simulink model "Simulation_Fahrmodell_v3_straight_line_R2024b"  (R2024b)
settings: Solver=ode14x  StartTime=0.0  StopTime=600  FixedStep=0.005  RelTol=1e-3
values from neighbouring files (symbols this model uses):
  bat = bat.computePack()    [DoE_main.m]    (also in DoE_main_sensitivity.m)
  cp = cp.computeP4Map(val_P4, 0, val_P4_DM, 0, 0)    [DoE_main.m]    (also in DoE_main_sensitivity.m = cp.computeP4Map(P4, E2, P4_DM, E3, E4))
  gb = gb.computeShiftMaps()    [DoE_main.m]    (also in DoE_main_sensitivity.m)
  P4 = cfgNum(cfg, 'P4', 0)    [DoE_main_sensitivity.m]    (also in PowertrainConfig.m = 0)
  P4_DM = cfgNum(cfg, 'P4_DM', 0)    [DoE_main_sensitivity.m]    (also in PowertrainConfig.m = 0)
  pt = pt.setupHybrid()    [DoE_main.m]    (also in DoE_main_sensitivity.m)
  veh = VehicleConfig()    [DoE_main.m]    (also in DoE_main_sensitivity.m)
undefined symbols (not defined in the file or in its folder): cp_Zelle_JpkgK, Ice_derfacLoadDecrease_MAP, Ice_derfacLoadIncrease_MAP, Ice_n_axis, Ice_relLoadMax_CUR_n, Ice_relLoadMax_CUR_val, Ice_rl_axis_norm, seconds, SKO_STREET_CHAL, SKO_WHEEL_TYP_CHAL, slip_pacejka, T_init_degC, Track, TT_sliced, use_turbo_model, v_Fzg_init_kmph
libraries: nesl_utility x15, fl_lib x9, simulink x4
(part 1 of 6)
settings Model: Creator=TZ555AA  LastModifiedBy=SHIKHAR TAKKE
settings DebuggingCC: SignalInfNanChecking=warning
settings RTWCC: GPUComputeCapability=3.5

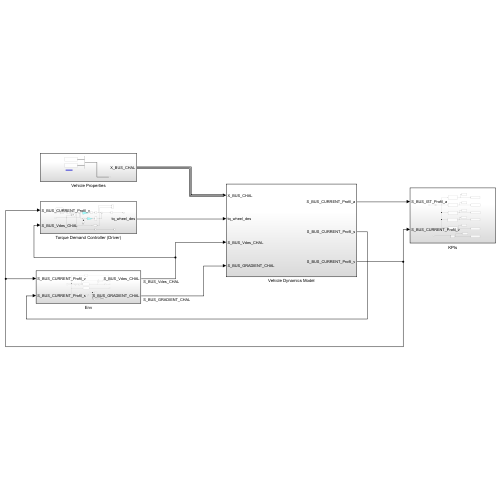
[thumbnail: Simulink's stored preview of the top-level diagram]
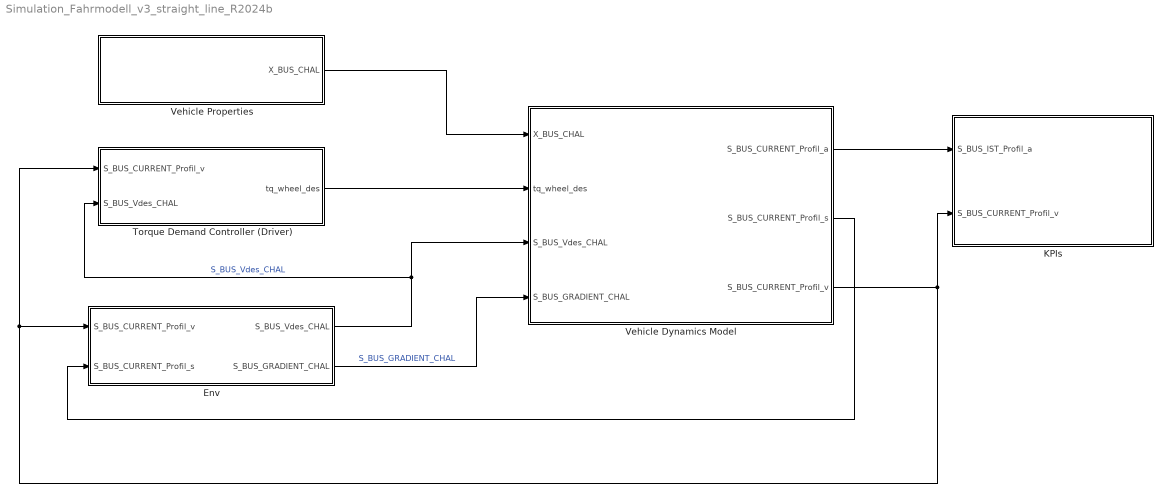
== system Simulation_Fahrmodell_v3_straight_line_R2024b ==
  Env : Subsystem
  KPIs : Subsystem
  Torque Demand Controller (Driver) : Subsystem
  "Vehicle Dynamics Model " : Subsystem
  Vehicle Properties : Subsystem
  wires:
  "Vehicle Dynamics Model "/1(S_BUS_CURRENT_Profil_a) -> KPIs/1(S_BUS_IST_Profil_a)
  "Vehicle Dynamics Model "/3(S_BUS_CURRENT_Profil_v) -> KPIs/2(S_BUS_CURRENT_Profil_v), Torque Demand Controller (Driver)/1(S_BUS_CURRENT_Profil_v), Env/1(S_BUS_CURRENT_Profil_v)
  "Vehicle Dynamics Model "/2(S_BUS_CURRENT_Profil_s) -> Env/2(S_BUS_CURRENT_Profil_s)
  Env/2(S_BUS_GRADIENT_CHAL) -> "Vehicle Dynamics Model "/4(S_BUS_GRADIENT_CHAL)  "S_BUS_GRADIENT_CHAL"
  Env/1(S_BUS_Vdes_CHAL) -> "Vehicle Dynamics Model "/3(S_BUS_Vdes_CHAL), Torque Demand Controller (Driver)/2(S_BUS_Vdes_CHAL)  "S_BUS_Vdes_CHAL"
  Torque Demand Controller (Driver)/1(tq_wheel_des) -> "Vehicle Dynamics Model "/2(tq_wheel_des)
  Vehicle Properties/1(X_BUS_CHAL) -> "Vehicle Dynamics Model "/1(X_BUS_CHAL)

== system Simulation_Fahrmodell_v3_straight_line_R2024b/Env ==
  S_BUS_CURRENT_Profil_v : Inport
  S_BUS_CURRENT_Profil_s : Inport  Port=2
  Bus Creator : BusCreator  Inputs=2
  Clock : Clock
  Constant : Constant  Value=seconds(TT_sliced.time(end))
  Display1 : Display
  Display3 : Display
  Gain : Gain
  Gain1 : Gain
  Gain2 : Gain  Gain=1/3.6
  Gain3 : Gain  Gain=3.6
  Gain4 : Gain
  Min : MinMax  Inputs=2
  Minus : Sum  Inputs=+-
  Nürburgring Simulation J. Siwig 469s (7m 49s) : Lookup_n-D  NumberOfTableDimensions=1  BreakpointsForDimension1=TT_sliced.s_m  Table=TT_sliced.v_Fzg_kmph  ExtrapMethod=Clip  UseLastTableValue=on  InternalRulePriority=Speed  RndMeth=Simplest
  Nürburgring Simulation J. Siwig 469s (7m 49s) time(s) : Lookup_n-D  NumberOfTableDimensions=1  BreakpointsForDimension1=TT_sliced.s_m  Table=seconds(TT_sliced.time)  ExtrapMethod=Clip  UseLastTableValue=on  InternalRulePriority=Speed  RndMeth=Simplest
  Nürburgring (M. Siesmann) : Subsystem
  Nürburgring (M. Siesmann) Steigung [deg] : Subsystem
  Scope : Scope  NumInputPorts=3
  Scope1 : Scope  NumInputPorts=2
  S_BUS_Vdes_CHAL : Outport
  S_BUS_GRADIENT_CHAL : Outport  Port=2
  wires:
  Gain3/1 -> Gain/1, Nürburgring (M. Siesmann)/2(v_ist_kmph)  "v_ist_kmph"
  Gain4/1 -> Gain3/1  "v_ist_mps"
  S_BUS_CURRENT_Profil_v/1 -> Gain4/1
  S_BUS_CURRENT_Profil_s/1 -> Nürburgring Simulation J. Siwig 469s (7m 49s)/1, Nürburgring (M. Siesmann)/1(s_m), Nürburgring Simulation J. Siwig 469s (7m 49s) time(s)/1, Nürburgring (M. Siesmann) Steigung [deg]/1(s_m)
  Nürburgring (M. Siesmann) Steigung [deg]/1(steigung_deg) -> S_BUS_GRADIENT_CHAL/1  "S_BUS_STEIGUNG_CHAL"
  Gain2/1 -> S_BUS_Vdes_CHAL/1
  Nürburgring (M. Siesmann)/1(v_soll_kmph) -> Gain2/1, Gain1/1  "[km/h]"
  Nürburgring Simulation J. Siwig 469s (7m 49s)/1 -> Scope/1  "MESSUNG v_Fzg_kmph"
  Gain/1 -> Scope/2  "SIM v_ist_kmph"
  Gain1/1 -> Scope/3  "SIM v_soll_kmph"
  Clock/1 -> Minus/2, Bus Creator/2, Display3/1  "SIM zeit"
  Min/1 -> Bus Creator/1, Minus/1, Display1/1  "MESSUNG zeit"
  Minus/1 -> Scope1/2  "DELTA zeit"
  Bus Creator/1 -> Scope1/1
  Constant/1 -> Min/2
  Nürburgring Simulation J. Siwig 469s (7m 49s) time(s)/1 -> Min/1  "MESSUNG zeit"

== system Simulation_Fahrmodell_v3_straight_line_R2024b/KPIs ==
  S_BUS_IST_Profil_a : Inport
  S_BUS_CURRENT_Profil_v : Inport  Port=2
  Display{1..5,7} (6 alike) : Display
  Gain : Gain  Gain=3.6
  MinMax Running Resettable1 : simulink/Math Operations/MinMax Running Resettable  Function=max  vinit=0
  To Workspace1 : ToWorkspace  VariableName=time_0_to_100  SampleTime=-1
      settings: MaxDataPoints=1
  To Workspace2 : ToWorkspace  VariableName=time_80_to_120  SampleTime=-1
      settings: MaxDataPoints=1
  To Workspace3 : ToWorkspace  VariableName=time_0_to_200  SampleTime=-1
      settings: MaxDataPoints=1
  To Workspace4 : ToWorkspace  VariableName=max_speed  SampleTime=-1
      settings: MaxDataPoints=1
  To Workspace5 : ToWorkspace  VariableName=max_launch_acc  SampleTime=-1
      settings: MaxDataPoints=1
  To Workspace6 : ToWorkspace  VariableName=time_60_to_120  SampleTime=-1
      settings: MaxDataPoints=1
  max speed : Subsystem
  time_0_to_100 : Subsystem
  time_0_to_200 : Subsystem
  time_60_to_120 : Subsystem
  time_80_to_120 : Subsystem
  wires:
  time_80_to_120/1(Out1) -> Display5/1, To Workspace2/1
  time_0_to_200/1(Out1) -> To Workspace3/1, Display4/1
  time_0_to_100/1(Out1) -> Display2/1, To Workspace1/1
  S_BUS_CURRENT_Profil_v/1 -> Gain/1
  S_BUS_IST_Profil_a/1 -> MinMax Running Resettable1/1
  MinMax Running Resettable1/1 -> Display7/1, To Workspace5/1
  max speed/1(u1) -> Display1/1, To Workspace4/1
  time_60_to_120/1(Out1) -> To Workspace6/1, Display3/1
  Gain/1 -> time_0_to_100/1(SIM v_ist_kmph), time_0_to_200/1(SIM v_ist_kmph), time_60_to_120/1(SIM v_ist_kmph), max speed/1(u), time_80_to_120/1(SIM v_ist_kmph)

== system Simulation_Fahrmodell_v3_straight_line_R2024b/Torque Demand Controller (Driver) ==
  S_BUS_CURRENT_Profil_v : Inport
  S_BUS_Vdes_CHAL : Inport  Port=2
  Drv_kmh2gradtqDriver_C Value: 300 : Gain  Gain=100
  Drv_kmh2tqDriver_C Value: 1500 : Gain  Gain=500
  Feedback I-Part at v=0 : Lookup_n-D  NumberOfTableDimensions=1  BreakpointsForDimension1="[-1 -0.0001  0  0.0001  1]"  Table="[0 0  1  0  0]"  InternalRulePriority=Speed  RndMeth=Simplest
  Gain : Gain
  Gain1 : Gain  Gain=0.005
  Gain2 : Gain  Gain=3.6
  Integrator : Integrator  LimitOutput=on  UpperSaturationLimit=2000  LowerSaturationLimit=-1200
  LowPass4Solver : TransferFcn  Denominator=[0.0001 1]
  MinMax : MinMax  Inputs=2
  Mux : Mux  Inputs=2
  Product : Product
  Saturation : Saturate  UpperLimit=7000  LowerLimit=-5000
  Saturation1 3000 : Saturate  UpperLimit=9000  LowerLimit=-5000
  Scope Ctrl. : Scope  NumInputPorts=2
  Scope kmh : Scope
  Sum : Sum  Inputs=|+-
  Sum1 : Sum  Inputs=|++
  Sum2 : Sum  Inputs=|+-
  Terminator : Terminator  Commented=on
  v_maxKmhEdr : Constant  Value=350
  tq_wheel_des : Outport  VectorParamsAs1DForOutWhenUnconnected=off
  wires:
  Mux/1 -> Scope kmh/1
  Gain2/1 -> MinMax/2
  MinMax/1 -> Gain/1, Sum/1, Mux/1  "Env_kmhVehDesLim"
  Gain1/1 -> Product/2  "Drv_kmhVehDesLim"
  Integrator/1 -> Gain1/1, Sum1/2, Scope Ctrl./2  "Drv_tqICtrlDrv[Nm]"
  Sum1/1 -> Saturation1 3000/1  "tqDrvWheelAxDesUnlim"
  S_BUS_Vdes_CHAL/1 -> Gain2/1
  Sum2/1 -> Drv_kmh2gradtqDriver_C Value: 300/1
  Saturation/1 -> Sum1/1, Scope Ctrl./1  "Drv_tqPCtrlDrv[Nm]"
  Feedback I-Part at v=0/1 -> Product/1
  v_maxKmhEdr/1 -> MinMax/1
  Sum/1 -> Sum2/1, Drv_kmh2tqDriver_C Value: 1500/1
  LowPass4Solver/1 -> Saturation/1
  Drv_kmh2tqDriver_C Value: 1500/1 -> LowPass4Solver/1
  S_BUS_CURRENT_Profil_v/1 -> Feedback I-Part at v=0/1, Sum/2, Mux/2
  Drv_kmh2gradtqDriver_C Value: 300/1 -> Integrator/1
  Saturation1 3000/1 -> tq_wheel_des/1  "tq_wheel_des"
  Product/1 -> Sum2/2
  Gain/1 -> Terminator/1  "Drv_kmhVehDesLim"

== system Simulation_Fahrmodell_v3_straight_line_R2024b/Vehicle Dynamics Model  ==
  X_BUS_CHAL : Inport
  tq_wheel_des : Inport  Port=2
  S_BUS_Vdes_CHAL : Inport  Port=3
  S_BUS_GRADIENT_CHAL : Inport  Port=4
  Bremsen : Subsystem
      mask Display: image('BremseVAHA_1.png');
  "Computation of Distance, Speed and Acceleration" : Subsystem
  Drivetrain : Subsystem
  Driving Resistance : Subsystem
  PI-Regler neu : Subsystem
  S_BUS_CURRENT_Profil_a : Outport
  S_BUS_CURRENT_Profil_s : Outport  Port=2
  S_BUS_CURRENT_Profil_v : Outport  Port=3
  wires:
  S_BUS_Vdes_CHAL/1 -> PI-Regler neu/1(S_BUS_Vdes_CHAL)
  X_BUS_CHAL/1 -> "Computation of Distance, Speed and Acceleration"/1(X_BUS_CHAL), Bremsen/1(X_BUS_CHAL), Drivetrain/2(X_BUS_CHAL1), Driving Resistance/1(X_BUS_CHAL)  "X_BUS_CHAL"
  S_BUS_GRADIENT_CHAL/1 -> Driving Resistance/3(BUS_STEIGUNG), Drivetrain/4(S_BUS_GRADIENT)
  Drivetrain/1(F_Lat_max (N)) -> "Computation of Distance, Speed and Acceleration"/2(F_Lat_max (N))  "F_Lat_max (N)"
  PI-Regler neu/1(Regelfaktor [-1 .. 1]) -> Drivetrain/1(Regelfaktor), Bremsen/2(Regelfaktor [-1 .. 1])
  "Computation of Distance, Speed and Acceleration"/1(S_BUS_IST_Profil_v) -> Driving Resistance/4(S_BUS_IST_Profil_v), Drivetrain/5(S_BUS_IST_Profil_v1), PI-Regler neu/2(S_BUS_IST_Profil_v), S_BUS_CURRENT_Profil_v/1  "S_BUS_IST_Profil_v"
  "Computation of Distance, Speed and Acceleration"/2(S_BUS_IST_Profil_s) -> S_BUS_CURRENT_Profil_s/1
  "Computation of Distance, Speed and Acceleration"/3(S_BUS_IST_Profil_a) -> Drivetrain/6(S_BUS_IST_Profil_a1), Driving Resistance/5(S_BUS_IST_Profil_a), S_BUS_CURRENT_Profil_a/1
  Bremsen/1(Bremskraft (N)) -> "Computation of Distance, Speed and Acceleration"/4(Bremskraft (N))  "Bremskraft (N)"
  tq_wheel_des/1 -> Drivetrain/3(tq_wheel_des)
  Drivetrain/2(M_m_Nm) -> Driving Resistance/2(M_m_Nm)
  Driving Resistance/1(FW_RSV (N)) -> "Computation of Distance, Speed and Acceleration"/3(FW_RSV (N))

== system Simulation_Fahrmodell_v3_straight_line_R2024b/Vehicle Properties ==
  note: Vehicle characteristics
  Bus Creator : BusCreator  Inputs=2
  Fzg.-Eigenschaften : Subsystem
  Systemkonstanten : Subsystem
  X_BUS_CHAL : Outport
  wires:
  Fzg.-Eigenschaften/1(M_BUS_EIG_CHAL) -> Bus Creator/2  "M_BUS_EIG_CHAL"
  Bus Creator/1 -> X_BUS_CHAL/1  "X_BUS_CHAL"
  Systemkonstanten/1(M_BUS_SKO) -> Bus Creator/1  "M_BUS_SKO"

== system Simulation_Fahrmodell_v3_straight_line_R2024b/Env/Nürburgring (M. Siesmann) ==
  s_m : Inport
  v_ist_kmph : Inport  Port=2
  Constant1 : Constant  Value=Track.RoundOnly.s_cum__m(end)
  Constant15 : Constant  Value=10000
  Display3 : Display
  Display4 : Display
  Fahrdynamik: Kurvenradius und Querbeschleunigung : Subsystem
  Fahrdynamik: Sollgeschwindigkeit (Kamm'scher Kreis) : Subsystem
  Low Pass Filter Amplitude = 1 Cut Off Freq = 3 KHz : TransferFcn  Commented=through  Denominator=[1/(2*pi*3000) 1]
  Min : MinMax  Inputs=2
  Relational Operator1 : RelationalOperator  OutDataTypeStr=boolean  RndMeth=Simplest  InputSameDT=off
  Scope : Scope  NumInputPorts=3
  Stop Simulation : Stop
  v max min : Subsystem
  vMax__km_per_h(s) vMax_Fwd : Lookup_n-D  Commented=on  NumberOfTableDimensions=1  BreakpointsForDimension1=Track.RoundOnly.s_cum__m  Table=Track.RoundOnly.vMax__km_per_h  InternalRulePriority=Speed  RndMeth=Simplest
  vMax__km_per_h(s) vMax_Fwd1 : Lookup_n-D  NumberOfTableDimensions=1  BreakpointsForDimension1=[0,2000]  Table=[300,300]  InternalRulePriority=Speed  RndMeth=Simplest
  v_soll_kmph : Outport
  wires:
  v_ist_kmph/1 -> Fahrdynamik: Kurvenradius und Querbeschleunigung/1(v_ist_kmph), Fahrdynamik: Sollgeschwindigkeit (Kamm'scher Kreis)/1(v_ist_kmph)
  Fahrdynamik: Sollgeschwindigkeit (Kamm'scher Kreis)/1(v_soll_kmph) -> Low Pass Filter Amplitude = 1 Cut Off Freq = 3 KHz/1
  Fahrdynamik: Kurvenradius und Querbeschleunigung/1(a_y_ist_mps2) -> Fahrdynamik: Sollgeschwindigkeit (Kamm'scher Kreis)/2(a_y_ist_mps2)
  Relational Operator1/1 -> Stop Simulation/1
  Constant15/1 -> Display4/1, Relational Operator1/2
  Min/1 -> v max min/1(In1), Scope/3  "v_soll_kmph END"
  Fahrdynamik: Kurvenradius und Querbeschleunigung/2(r_kurven_m) -> Fahrdynamik: Sollgeschwindigkeit (Kamm'scher Kreis)/3(r_kurven_m)
  v max min/1(Out1) -> v_soll_kmph/1
  s_m/1 -> vMax__km_per_h(s) vMax_Fwd1/1, Fahrdynamik: Kurvenradius und Querbeschleunigung/2(s_m), Display3/1, Relational Operator1/1
  Low Pass Filter Amplitude = 1 Cut Off Freq = 3 KHz/1 -> Scope/2, Min/2  "v_soll_kmph FDyn"
  vMax__km_per_h(s) vMax_Fwd1/1 -> Min/1, Scope/1  "v_soll_kmph 3SIM"

== system Simulation_Fahrmodell_v3_straight_line_R2024b/Env/Nürburgring (M. Siesmann) Steigung [deg] ==
  s_m : Inport
  Agl_Elevation__deg(s_cum_m) : Lookup_n-D  Commented=on  NumberOfTableDimensions=1  BreakpointsForDimension1=Track.RoundOnly.s_cum__m  Table=Track.RoundOnly.Agl_Elevation__deg  InternalRulePriority=Speed  RndMeth=Simplest
  Agl_Elevation__deg(s_cum_m)1 : Lookup_n-D  NumberOfTableDimensions=1  BreakpointsForDimension1=[0,2000]  Table=[0,0]  InternalRulePriority=Speed  RndMeth=Simplest
  steigung_deg : Outport
  wires:
  Agl_Elevation__deg(s_cum_m)1/1 -> steigung_deg/1  "steigung_deg"
  s_m/1 -> Agl_Elevation__deg(s_cum_m)1/1

== system Simulation_Fahrmodell_v3_straight_line_R2024b/KPIs/max speed ==
  u : Inport
  R : Inport  Port=2
  Add : Sum  Inputs=+-
  Compare To Constant : simulink/Logic and Bit Operations/Compare To Constant  relop===  const=0  OutDataTypeStr=boolean
  Compare To Constant1 : simulink/Logic and Bit Operations/Compare To Constant  relop=>  const=35  OutDataTypeStr=boolean
  Constant : Constant
  Delay : Delay  InitialCondition=0
  Display6 : Display
  MinMax Running Resettable : simulink/Math Operations/MinMax Running Resettable  Function=max  vinit=0
  Stop Simulation : Stop
  Switch : Switch  Criteria=u2 > Threshold  SaturateOnIntegerOverflow=off  InputSameDT=off
  u1 : Outport
  wires:
  MinMax Running Resettable/1 -> Compare To Constant1/1, Add/1, Delay/1, u1/1
  Compare To Constant/1 -> Stop Simulation/1, Display6/1
  Delay/1 -> Switch/1
  Compare To Constant1/1 -> Switch/2
  Add/1 -> Compare To Constant/1
  Constant/1 -> Switch/3
  Switch/1 -> Add/2
  u/1 -> MinMax Running Resettable/1
  R/1 -> MinMax Running Resettable/2

== system Simulation_Fahrmodell_v3_straight_line_R2024b/KPIs/time_0_to_100 ==
  SIM v_ist_kmph : Inport
  Clock : Clock
      settings: Decimation=100
  Constant : Constant
  Constant1 : Constant  Value=0
  Switch : Switch  Threshold=100  SaturateOnIntegerOverflow=off  InputSameDT=off
  Triggered Subsystem : Subsystem  TreatAsAtomicUnit=on
  Out1 : Outport
  wires:
  Constant/1 -> Switch/1
  SIM v_ist_kmph/1 -> Switch/2
  Switch/1 -> Triggered Subsystem/Trigger
  Clock/1 -> Triggered Subsystem/1(In1)
  Constant1/1 -> Switch/3
  Triggered Subsystem/1(Out1) -> Out1/1

== system Simulation_Fahrmodell_v3_straight_line_R2024b/KPIs/time_0_to_200 ==
  SIM v_ist_kmph : Inport
  Clock : Clock
      settings: Decimation=100
  Constant : Constant
  Constant1 : Constant  Value=0
  Switch : Switch  Threshold=200  SaturateOnIntegerOverflow=off  InputSameDT=off
  Triggered Subsystem : Subsystem  TreatAsAtomicUnit=on
  Out1 : Outport
  wires:
  Triggered Subsystem/1(Out1) -> Out1/1
  Constant1/1 -> Switch/3
  Clock/1 -> Triggered Subsystem/1(In1)
  Switch/1 -> Triggered Subsystem/Trigger
  SIM v_ist_kmph/1 -> Switch/2
  Constant/1 -> Switch/1

== system Simulation_Fahrmodell_v3_straight_line_R2024b/KPIs/time_60_to_120 ==
  SIM v_ist_kmph : Inport
  Add : Sum  Inputs=+-
  time_0_to_120 : Subsystem
  time_0_to_60 : Subsystem
  Out1 : Outport
  wires:
  Add/1 -> Out1/1
  time_0_to_120/1(Out1) -> Add/1
  time_0_to_60/1(Out1) -> Add/2
  SIM v_ist_kmph/1 -> time_0_to_60/1(In1), time_0_to_120/1(In1)

== system Simulation_Fahrmodell_v3_straight_line_R2024b/KPIs/time_80_to_120 ==
  SIM v_ist_kmph : Inport
  Add : Sum  Inputs=+-
  time_0_to_120 : Subsystem
  time_0_to_80 : Subsystem
  Out1 : Outport
  wires:
  SIM v_ist_kmph/1 -> time_0_to_120/1(In1), time_0_to_80/1(In1)
  time_0_to_80/1(Out1) -> Add/2
  time_0_to_120/1(Out1) -> Add/1
  Add/1 -> Out1/1

== system Simulation_Fahrmodell_v3_straight_line_R2024b/Vehicle Dynamics Model /Bremsen ==
  X_BUS_CHAL : Inport
  Regelfaktor [-1 .. 1] : Inport  Port=2
  Bremskraftfaktor abh. Bremspedalposition : Lookup_n-D  NumberOfTableDimensions=1  BreakpointsForDimension1=[0, 0.2, 0.4, 0.6, 0.8, 1]  Table=[0, 1, 2, 4, 6.5, 11]  InternalRulePriority=Speed  RndMeth=Simplest
  Bremspedal: Regelfaktor < 0 : MinMax  Inputs=2
  Bus Selector : BusSelector  OutputSignals=M_BUS_EIG_CHAL.S_BUS_EIG_GEW_CHAL,M_BUS_SKO.SKO_BRAKE
  Constant1 : Constant  Value=0
  Display1 : Display
  Display2 : Display
  Display3 : Display
  "Negieren, sodass positiv" : Gain  Gain=-1
  Product2 : Product  Inputs=3
  Scope1 : Scope  NumInputPorts=3
  Verstärkungsfaktor : Constant  Value=1.072
  Bremskraft (N) : Outport
  wires:
  Verstärkungsfaktor/1 -> Product2/2
  Product2/1 -> Scope1/3, Display1/1, Bremskraft (N)/1  "Bremskraft (N)"
  Bremskraftfaktor abh. Bremspedalposition/1 -> Scope1/2, Product2/1
  X_BUS_CHAL/1 -> Bus Selector/1  "X_BUS_CHAL"
  Bus Selector/1 -> Product2/3, Display2/1  "<S_BUS_EIG_GEW_CHAL>"
  Regelfaktor [-1 .. 1]/1 -> Bremspedal: Regelfaktor < 0/1
  "Negieren, sodass positiv"/1 -> Display3/1, Bremskraftfaktor abh. Bremspedalposition/1, Scope1/1
  Constant1/1 -> Bremspedal: Regelfaktor < 0/2
  Bremspedal: Regelfaktor < 0/1 -> "Negieren, sodass positiv"/1

== system Simulation_Fahrmodell_v3_straight_line_R2024b/Vehicle Dynamics Model /Computation of Distance, Speed and Acceleration ==
  X_BUS_CHAL : Inport
  F_Lat_max (N) : Inport  Port=2
  FW_RSV (N) : Inport  Port=3
  Bremskraft (N) : Inport  Port=4
  Bus Selector : BusSelector  OutputSignals=M_BUS_EIG_CHAL.S_BUS_EIG_GEW_CHAL
  Constant : Constant  Value=v_Fzg_init_kmph
  Delay : Delay  DelayLength=1
  Display : Display
  Divide3 : Product  Inputs=*/
  Integrator1 : Integrator  LimitOutput=on  LowerSaturationLimit=0
  Max : MinMax  Function=max  Inputs=2
  Start-Geschwindigkeit Init km/h (s. Init-Datei) : Integrator  InitialCondition=35/3.6  LimitOutput=on  LowerSaturationLimit=0
  Start-Geschwindigkeit Init km/h (s. Init-Datei)1 : Integrator  Commented=on  InitialCondition=v_Fzg_init_kmph/3.6  LimitOutput=on  LowerSaturationLimit=0
  Sum2 : Sum  Inputs=+-
  S_BUS_IST_Profil_v : Outport
  S_BUS_IST_Profil_s : Outport  Port=2
  S_BUS_IST_Profil_a : Outport  Port=3
  tag scope: S_BUS_IST_Profil_a=global
  wires:
  FW_RSV (N)/1 -> Max/1
  F_Lat_max (N)/1 -> Sum2/1
  Bremskraft (N)/1 -> Max/2
  Bus Selector/1 -> Divide3/2  "<S_BUS_EIG_GEW_CHAL>"
  Start-Geschwindigkeit Init km/h (s. Init-Datei)/1 -> Integrator1/1, S_BUS_IST_Profil_v/1  "S_BUS_IST_Profil_v"
  Max/1 -> Sum2/2  "Fahrwiderstaende (N)"
  X_BUS_CHAL/1 -> Bus Selector/1
  Divide3/1 -> Delay/1, Start-Geschwindigkeit Init km/h (s. Init-Datei)/1  "S_BUS_IST_Profil_a"
  Sum2/1 -> Divide3/1  "\"Beschleunigungs\"-Kraft"
  Integrator1/1 -> S_BUS_IST_Profil_s/1  "S_BUS_IST_Profil_s"
  Constant/1 -> Display/1
  Delay/1 -> [S_BUS_IST_Profil_a], S_BUS_IST_Profil_a/1

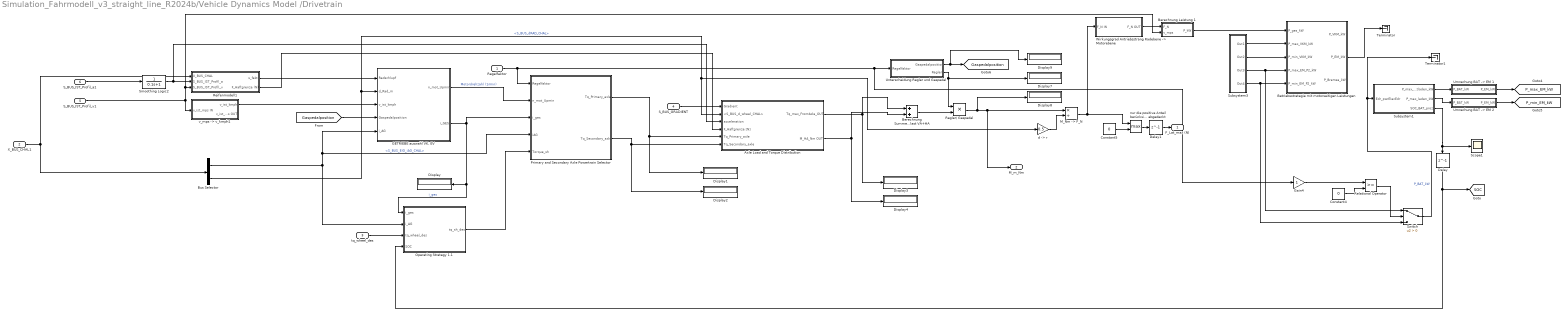
== system Simulation_Fahrmodell_v3_straight_line_R2024b/Vehicle Dynamics Model /Drivetrain ==
  Regelfaktor : Inport
  X_BUS_CHAL1 : Inport  Port=2
  tq_wheel_des : Inport  Port=3
  S_BUS_GRADIENT : Inport  Port=4
  S_BUS_IST_Profil_v1 : Inport  Port=5
  S_BUS_IST_Profil_a1 : Inport  Port=6
  "Axle Load and Torque Distribution " : Subsystem
  Berechnung Summenradlast VA+HA : Sum
  Berechnung Leistung 1 : Subsystem
  Betriebsstrategie mit motorseitigen Leistungen : Subsystem
  Bus Selector : BusSelector  OutputSignals=M_BUS_EIG_CHAL.S_BUS_EIG_iAG_CHAL,M_BUS_EIG_CHAL.S_BUS_dRAD_CHAL
  Constant4 : Constant  Value=0
  Constant5 : Constant  Value=0
  Delay : Delay  DelayLength=1
  Delay1 : Delay  DelayLength=1  InputProcessing=Columns as channels (frame based)
  Display{,1..4,7..9} (8 alike) : Display
  "GETRIEBE auswahl VK, EV" : Subsystem  VariantControl=Choice
  Gain4 : Gain
  "M_Nm -> F_N" : Product  Inputs=*/
  Operating Strategy 1.1 : Subsystem
  Primary and Secondary Axle Powertrain Selector : Subsystem
  Regler/ Gaspedal : Product
  Reifenmodell1 : Subsystem
  Relational Operator : RelationalOperator  OutDataTypeStr=boolean  RndMeth=Simplest  InputSameDT=off
  Scope1 : Scope
  Smoothing Logic2 : TransferFcn  Denominator=[0.1 1]
  Subsystem1 : Subsystem
  Subsystem3 : Subsystem
  Switch : Switch  Criteria=u2 > Threshold  SaturateOnIntegerOverflow=off  InputSameDT=off
  Terminator : Terminator
  Terminator1 : Terminator
  "Umrechung BAT -> EM 1" : Subsystem
  "Umrechung BAT -> EM 2" : Subsystem
  Unterscheidung Regler und Gaspedal : Subsystem
  "Wirkungsgrad Antriebsstrang Radebene -> Motorebene" : Subsystem
  "d -> r" : Gain  Gain=0.5
  nur die positive Anteil berücksichtigt; die negative Anteil wurde bereits mit Bremsen abgedeckt : MinMax  Function=max  Inputs=2
  "v_mps -> v_kmph1" : Subsystem
  F_Lat_max (N) : Outport
  M_m_Nm : Outport  Port=2
  tag scope: Gaspedalposition=global, P_max_EM_kW=global, P_min_EM_kW=global, SOC=global
  wires:
  Reifenmodell1/1(s_fakt) -> "GETRIEBE auswahl VK, EV"/1(Radschlupf)
  "v_mps -> v_kmph1"/1(v_ist_kmph) -> "GETRIEBE auswahl VK, EV"/3(v_ist_kmph)
  X_BUS_CHAL1/1 -> Bus Selector/1, Reifenmodell1/1(X_BUS_CHAL)
  S_BUS_IST_Profil_a1/1 -> Smoothing Logic2/1
  [Gaspedalposition] -> "GETRIEBE auswahl VK, EV"/4(Gaspedalposition)
  Smoothing Logic2/1 -> "Axle Load and Torque Distribution "/3(acceleration), Reifenmodell1/2(S_BUS_IST_Profil_a)
  Unterscheidung Regler und Gaspedal/1(Gaspedalposition) -> Display9/1, [Gaspedalposition]
  "M_Nm -> F_N"/1 -> nur die positive Anteil berücksichtigt; die negative Anteil wurde bereits mit Bremsen abgedeckt/1, "Wirkungsgrad Antriebsstrang Radebene -> Motorebene"/1(F_N IN)
  Unterscheidung Regler und Gaspedal/2(Regler) -> Display7/1, Regler/ Gaspedal/1
  Constant5/1 -> nur die positive Anteil berücksichtigt; die negative Anteil wurde bereits mit Bremsen abgedeckt/2
  Regler/ Gaspedal/1 -> Display8/1, M_m_Nm/1, "M_Nm -> F_N"/1
  Berechnung Summenradlast VA+HA/1 -> Regler/ Gaspedal/2
  nur die positive Anteil berücksichtigt; die negative Anteil wurde bereits mit Bremsen abgedeckt/1 -> Delay1/1
  "d -> r"/1 -> "M_Nm -> F_N"/2
  "Wirkungsgrad Antriebsstrang Radebene -> Motorebene"/1(F_N OUT) -> Berechnung Leistung 1/1(F_N)
  S_BUS_IST_Profil_v1/1 -> Berechnung Leistung 1/2(v_mps), Reifenmodell1/3(S_BUS_IST_Profil_v), "v_mps -> v_kmph1"/1(v_ist_mps IN)
  Berechnung Leistung 1/1(P_kW) -> Betriebsstrategie mit motorseitigen Leistungen/1(P_ges_kW)
  "GETRIEBE auswahl VK, EV"/1(n_mot_Upmin) -> Primary and Secondary Axle Powertrain Selector/2(n_mot_Upmin)  "Motordrehzahl (1/min)"
  "GETRIEBE auswahl VK, EV"/2(i_GES) -> Operating Strategy 1.1/1(i_ges), Display/1, Primary and Secondary Axle Powertrain Selector/3(i_ges)  "i_ges"
  Betriebsstrategie mit motorseitigen Leistungen/2(P_EM_kW) -> Terminator/1
  Subsystem1/2(P_max_laden_kW) -> "Umrechung BAT -> EM 2"/1(P_BAT_kW)
  Subsystem1/1(P_max_entladen_kW) -> "Umrechung BAT -> EM 1"/1(P_BAT_kW)
  "Umrechung BAT -> EM 1"/1(P_EM_kW) -> [P_max_EM_kW]
  "Umrechung BAT -> EM 2"/1(P_EM_kW) -> [P_min_EM_kW]
  Subsystem3/1(Out1) -> Betriebsstrategie mit motorseitigen Leistungen/2(P_max_VKM_kW)
  Subsystem3/2(Out2) -> Betriebsstrategie mit motorseitigen Leistungen/3(P_min_VKM_kW)
  Subsystem3/3(Out3) -> Switch/1, Betriebsstrategie mit motorseitigen Leistungen/4(P_max_EM_P2_kW)
  Subsystem3/4(Out4) -> Switch/3, Betriebsstrategie mit motorseitigen Leistungen/5(P_min_EM_P2_kW)
  Bus Selector/2 -> "Axle Load and Torque Distribution "/2(<S_BUS_d_wheel_CHAL>), "d -> r"/1, "GETRIEBE auswahl VK, EV"/2(d_Rad_m)  "<S_BUS_dRAD_CHAL>"
  Bus Selector/1 -> Operating Strategy 1.1/2(i_AG), Primary and Secondary Axle Powertrain Selector/4(iAG), "GETRIEBE auswahl VK, EV"/5(i_AG)  "<S_BUS_EIG_iAG_CHAL>"
  Primary and Secondary Axle Powertrain Selector/1(Tq_Primary_axle) -> "Axle Load and Torque Distribution "/5(Tq_Primary_axle), Display1/1
  Primary and Secondary Axle Powertrain Selector/2(Tq_Secondary_axle) -> "Axle Load and Torque Distribution "/6(Tq_Secondary_axle), Display2/1
  Subsystem1/3(SOC_BAT_proz) -> Delay/1, Scope1/1
  tq_wheel_des/1 -> Operating Strategy 1.1/3(tq_wheel_des)
  Operating Strategy 1.1/1(tq_sh_des) -> Primary and Secondary Axle Powertrain Selector/5(Torque_sh)
  Regelfaktor/1 -> Gain4/1, Unterscheidung Regler und Gaspedal/1(Regelfaktor), Primary and Secondary Axle Powertrain Selector/1(Regelfaktor)
  Relational Operator/1 -> Switch/2
  Constant4/1 -> Relational Operator/2
  Switch/1 -> Terminator1/1, Subsystem1/1(Edr_pwrElecEdr)  "P_BAT_kW"
  Gain4/1 -> Relational Operator/1
  Delay/1 -> [SOC], Operating Strategy 1.1/4(SOC)
  Delay1/1 -> F_Lat_max (N)/1
  "Axle Load and Torque Distribution "/2(M_HA_Nm OUT) -> Berechnung Summenradlast VA+HA/2, Display4/1
  "Axle Load and Torque Distribution "/1(Tq_max_FrontAxle_OUT) -> Berechnung Summenradlast VA+HA/1, Display3/1
  S_BUS_GRADIENT/1 -> "Axle Load and Torque Distribution "/1(Gradient)
  Reifenmodell1/2(F_Haftgrenze (N)) -> "Axle Load and Torque Distribution "/4(F_Haftgrenze [N])

== system Simulation_Fahrmodell_v3_straight_line_R2024b/Vehicle Dynamics Model /Driving Resistance ==
  X_BUS_CHAL : Inport
  M_m_Nm : Inport  Port=2
  BUS_STEIGUNG : Inport  Port=3
  S_BUS_IST_Profil_v : Inport  Port=4
  S_BUS_IST_Profil_a : Inport  Port=5
  Delay : Delay  DelayLength=1
  Divide : Product  Inputs=*/
  Fahrwiderstand : Subsystem
  Minus : Sum  Inputs=+-
  Scope : Scope
  Scope4 : Scope  NumInputPorts=2
  Subsystem : Subsystem
  Terminator : Terminator
  FW_RSV (N) : Outport
  wires:
  Minus/1 -> Divide/1
  X_BUS_CHAL/1 -> Subsystem/1(X_BUS_CHAL), Fahrwiderstand/1(X_BUS_CHAL)
  BUS_STEIGUNG/1 -> Subsystem/2(BUS_STEIGUNG), Fahrwiderstand/2(BUS_STEIGUNG)
  S_BUS_IST_Profil_v/1 -> Fahrwiderstand/3(S_BUS_IST_Profil_v), Scope4/2, Scope4/1, Minus/1, Delay/1
  Delay/1 -> Divide/2, Minus/2
  Divide/1 -> Scope/1
  Fahrwiderstand/2(S_BUS_FLST_Wges) -> Terminator/1  "FW_GES (N)"
  Fahrwiderstand/1(S_BUS_FLST_Wrls) -> FW_RSV (N)/1  "FW_RSV (N)"
  S_BUS_IST_Profil_a/1 -> Fahrwiderstand/4(S_BUS_IST_Profil_a)
  M_m_Nm/1 -> Subsystem/3(M_m_Nm)

== system Simulation_Fahrmodell_v3_straight_line_R2024b/Vehicle Dynamics Model /PI-Regler neu ==
  S_BUS_Vdes_CHAL : Inport
  S_BUS_IST_Profil_v : Inport  Port=2
  Add : Sum
  Bus Creator : BusCreator  Inputs=3
  Display : Display
  Gain : Gain  Gain=5
  Gain1 : Gain  Gain=10
  Integrator : Integrator  LimitOutput=on  UpperSaturationLimit=1  LowerSaturationLimit=-0.5
  Limit output : Saturate  UpperLimit=1  LowerLimit=-1
  Saturation1 : Saturate  UpperLimit=1  LowerLimit=-1
  Scope : Scope  NumInputPorts=4
  Scope1 : Scope
  Smoothing function2 : TransferFcn  Denominator=[0.01 1]
  Sum3 : Sum  Inputs=-+
  Regelfaktor [-1 .. 1] : Outport
  wires:
  Sum3/1 -> Scope/1, Gain/1, Gain1/1, Display/1  "Regeldifferenz"
  Integrator/1 -> Scope/3, Add/2
  Add/1 -> Smoothing function2/1, Bus Creator/1
  Gain/1 -> Integrator/1
  Saturation1/1 -> Scope/2, Add/1
  Bus Creator/1 -> Scope/4
  Limit output/1 -> Bus Creator/2, Scope1/1, Regelfaktor [-1 .. 1]/1
  Gain1/1 -> Saturation1/1
  Smoothing function2/1 -> Limit output/1
  S_BUS_IST_Profil_v/1 -> Sum3/1
  S_BUS_Vdes_CHAL/1 -> Sum3/2

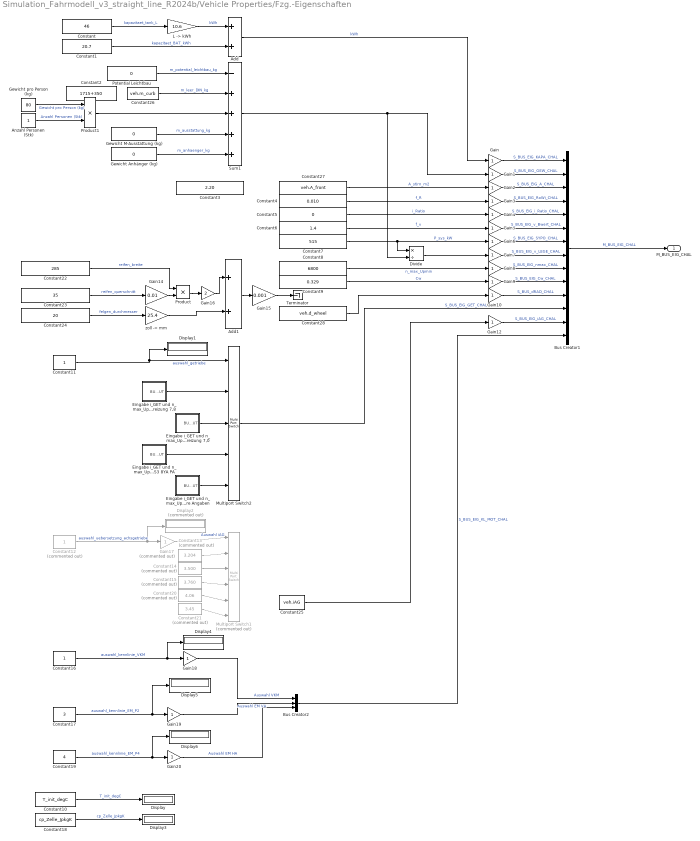
== system Simulation_Fahrmodell_v3_straight_line_R2024b/Vehicle Properties/Fzg.-Eigenschaften ==
  Add : Sum
  Add1 : Sum
  Anzahl Personen (Stk) : Constant
  Bus Creator1 : BusCreator  Inputs=14
  Bus Creator2 : BusCreator  Inputs=3
  Constant : Constant  Value=46
  Constant1 : Constant  Value=20.7
  Constant10 : Constant  Value=T_init_degC
  Constant11 : Constant
  Constant12 : Constant  Commented=on
  Constant13 : Constant  Commented=on  Value=3.204
  Constant14 : Constant  Commented=on  Value=3.500
  Constant15 : Constant  Commented=on  Value=3.760
  Constant16 : Constant
  Constant17 : Constant  Value=3
  Constant18 : Constant  Value=cp_Zelle_JpkgK
  Constant19 : Constant  Value=4
  Constant2 : Constant  Value=1715+350
  Constant20 : Constant  Commented=on  Value=4.06
  Constant21 : Constant  Commented=on  Value=3.45
  Constant22 : Constant  Value=285
  Constant23 : Constant  Value=35
  Constant24 : Constant  Value=20
  Constant25 : Constant  Value=veh.iAG
  Constant26 : Constant  Value=veh.m_curb
  Constant27 : Constant  Value=veh.A_front
  Constant28 : Constant  Value=veh.d_wheel
  Constant3 : Constant  Value=2.20
  Constant4 : Constant  Value=0.010
  Constant5 : Constant  Value=0
  Constant6 : Constant  Value=1.4
  Constant7 : Constant  Value=515
  Constant8 : Constant  Value=6800
  Constant9 : Constant  Value=0.329
  Display{,1,3..6} (6 alike) : Display
  Display2 : Display  Commented=on
  Divide : Product  Inputs=*/
  Eingabe i_GET und n_max_Upmin Andere Angaben : Subsystem  mask{n_max_Upmin_G1=6800, i_G1=4.714, n_max_Upmin_G2=6800, i_G2=3.143, n_max_Upmin_G3=6800, i_G3=2.106, n_max_Upmin_G4=6800, i_G4=1.667, n_max_Upmin_G5=6800, i_G5=1.285, n_max_Upmin_G6=6800, i_G6=1.000, n_max_Upmin_G7=6200, i_G7=0.839, n_max_Upmin_G8=6200, i_G8=0.667}
      mask DialogControl ParameterGroupVar Prompt: Getriebe - Max. Drehzahl und Übersetzung
      mask DialogControl Control2 Prompt: Gang
      mask DialogControl Control3 Prompt: n_max [U/min]
      mask DialogControl Control4 Prompt: i_Gang
      mask DialogControl G1 Prompt: 1
      mask DialogControl G2 Prompt: 2
      mask DialogControl G3 Prompt: 3
      mask DialogControl G4 Prompt: 4
      mask DialogControl G5 Prompt: 5
      mask DialogControl G6 Prompt: 6
      mask DialogControl G7 Prompt: 7
      mask DialogControl G8 Prompt: 8
  Eingabe i_GET und n_max_Upmin Audi RS3 8YA PA : Subsystem  mask{n_max_Upmin_G1=6800, i_G1=3.56, n_max_Upmin_G2=6800, i_G2=2.53, n_max_Upmin_G3=6800, i_G3=1.68, n_max_Upmin_G4=6800, i_G4=1.02, n_max_Upmin_G5=6800, i_G5=0.79, n_max_Upmin_G6=6800, i_G6=0.76, n_max_Upmin_G7=9999, i_G7=0.63, n_max_Upmin_G8=9999, i_G8=0.63}
      mask DialogControl ParameterGroupVar Prompt: Getriebe - Max. Drehzahl und Übersetzung
      mask DialogControl Control2 Prompt: Gang
      mask DialogControl Control3 Prompt: n_max [U/min]
      mask DialogControl Control4 Prompt: i_Gang
      mask DialogControl G1 Prompt: 1
      mask DialogControl G2 Prompt: 2
      mask DialogControl G3 Prompt: 3
      mask DialogControl G4 Prompt: 4
      mask DialogControl G5 Prompt: 5
      mask DialogControl G6 Prompt: 6
      mask DialogControl G7 Prompt: 7
      mask DialogControl G8 Prompt: 8
  Eingabe i_GET und n_max_Upmin Spreizung 7,0 : Subsystem  mask{n_max_Upmin_G1=6800, i_G1=4.714, n_max_Upmin_G2=6800, i_G2=3.143, n_max_Upmin_G3=6800, i_G3=2.106, n_max_Upmin_G4=6800, i_G4=1.667, n_max_Upmin_G5=6800, i_G5=1.285, n_max_Upmin_G6=6800, i_G6=1.000, n_max_Upmin_G7=6200, i_G7=0.839, n_max_Upmin_G8=6200, i_G8=0.667}
      mask DialogControl ParameterGroupVar Prompt: Getriebe - Max. Drehzahl und Übersetzung
      mask DialogControl Control2 Prompt: Gang
      mask DialogControl Control3 Prompt: n_max [U/min]
      mask DialogControl Control4 Prompt: i_Gang
      mask DialogControl G1 Prompt: 1
      mask DialogControl G2 Prompt: 2
      mask DialogControl G3 Prompt: 3
      mask DialogControl G4 Prompt: 4
      mask DialogControl G5 Prompt: 5
      mask DialogControl G6 Prompt: 6
      mask DialogControl G7 Prompt: 7
      mask DialogControl G8 Prompt: 8
  Eingabe i_GET und n_max_Upmin Spreizung 7,8 : Subsystem  mask{n_max_Upmin_G1=6800, i_G1=5.000, n_max_Upmin_G2=6800, i_G2=3.200, n_max_Upmin_G3=6800, i_G3=2.143, n_max_Upmin_G4=6800, i_G4=1.720, n_max_Upmin_G5=6800, i_G5=1.313, n_max_Upmin_G6=6800, i_G6=1.000, n_max_Upmin_G7=6200, i_G7=0.823, n_max_Upmin_G8=6200, i_G8=0.640}
      mask DialogControl ParameterGroupVar Prompt: Getriebe - Max. Drehzahl und Übersetzung
      mask DialogControl Control2 Prompt: Gang
      mask DialogControl Control3 Prompt: n_max [U/min]
      mask DialogControl Control4 Prompt: i_Gang
      mask DialogControl G1 Prompt: 1
      mask DialogControl G2 Prompt: 2
      mask DialogControl G3 Prompt: 3
      mask DialogControl G4 Prompt: 4
      mask DialogControl G5 Prompt: 5
      mask DialogControl G6 Prompt: 6
      mask DialogControl G7 Prompt: 7
      mask DialogControl G8 Prompt: 8
  Gain{,1..10,12,18..20} (15 alike) : Gain
  Gain14 : Gain  Gain=0.01
  Gain15 : Gain  Gain=0.001
  Gain16 : Gain  Gain=2
  Gain17 : Gain  Commented=on
  Gewicht Anhänger (kg) : Constant  Value=0
  Gewicht M-Ausstattung (kg) : Constant  Value=0
  Gewicht pro Person (kg) : Constant  Value=80
  "L -> kWh" : Gain  Gain=10.6
  Multiport Switch1 : MultiPortSwitch  Commented=on  Inputs=5  SaturateOnIntegerOverflow=off  InputSameDT=off
  Multiport Switch2 : MultiPortSwitch  Inputs=4  SaturateOnIntegerOverflow=off  InputSameDT=off
  Potential Leichtbau : Constant  Value=0
  Product : Product
  Product1 : Product
  Sum1 : Sum  Inputs=-++++
  Terminator : Terminator
  "zoll -> mm" : Gain  Gain=25.4
  M_BUS_EIG_CHAL : Outport
  wires:
  Gain/1 -> Bus Creator1/1  "S_BUS_EIG_KAPA_CHAL"
  Gain1/1 -> Bus Creator1/2  "S_BUS_EIG_GEW_CHAL"
  Gain2/1 -> Bus Creator1/3  "S_BUS_EIG_A_CHAL"
  Gain3/1 -> Bus Creator1/4  "S_BUS_EIG_RoWi_CHAL"
  Gain4/1 -> Bus Creator1/5  "S_BUS_EIG_i_Ratio_CHAL"
  Gain5/1 -> Bus Creator1/6  "S_BUS_EIG_v_Bwert_CHAL"
  Gain6/1 -> Bus Creator1/7  "S_BUS_EIG_SYPO_CHAL"
  Gain7/1 -> Bus Creator1/8  "S_BUS_EIG_v_LEGE_CHAL"
  Gain8/1 -> Bus Creator1/9  "S_BUS_EIG_nmax_CHAL"
  Gain9/1 -> Bus Creator1/10  "S_BUS_EIG_Cw_CHAL"
  Gain10/1 -> Bus Creator1/11  "S_BUS_dRAD_CHAL"
  Multiport Switch2/1 -> Bus Creator1/12  "S_BUS_EIG_GET_CHAL"
  Gain12/1 -> Bus Creator1/13  "S_BUS_EIG_iAG_CHAL"
  Bus Creator2/1 -> Bus Creator1/14  "S_BUS_EIG_KL_MOT_CHAL"
  Bus Creator1/1 -> M_BUS_EIG_CHAL/1  "M_BUS_EIG_CHAL"
  Add/1 -> Gain/1  "kWh"
  Constant/1 -> "L -> kWh"/1  "kapazitaet_tank_L"
  "L -> kWh"/1 -> Add/1  "kWh"
  Constant1/1 -> Add/2  "kapazitaet_BAT_kWh"
  Gewicht M-Ausstattung (kg)/1 -> Sum1/4  "m_ausstattung_kg"
  Product1/1 -> Sum1/3
  Anzahl Personen (Stk)/1 -> Product1/2  "Anzahl Personen (Stk)"
  Gewicht Anhänger (kg)/1 -> Sum1/5  "m_anhaenger_kg"
  Sum1/1 -> Divide/2, Gain1/1
  Constant26/1 -> Sum1/2  "m_leer_DIN_kg"
  Potential Leichtbau/1 -> Sum1/1  "m_potential_leichtbau_kg"
  Gewicht pro Person (kg)/1 -> Product1/1  "Gewicht pro Person (kg)"
  Constant6/1 -> Gain5/1  "f_v"
  Constant8/1 -> Gain8/1  "n_max_Upmin"
  Constant5/1 -> Gain4/1  "i_Ratio"
  Constant9/1 -> Gain9/1  "Cw"
  Constant7/1 -> Divide/1, Gain6/1  "P_sys_kW"
  Constant27/1 -> Gain2/1  "A_stirn_m2"
  Divide/1 -> Gain7/1
  Constant4/1 -> Gain3/1  "f_R"
  Constant24/1 -> "zoll -> mm"/1  "felgen_durchmesser"
  Product/1 -> Gain16/1
  Add1/1 -> Gain15/1
  "zoll -> mm"/1 -> Add1/2
  Gain16/1 -> Add1/1
  Constant22/1 -> Product/1  "reifen_breite"
  Gain14/1 -> Product/2
  Constant23/1 -> Gain14/1  "reifen_querschnitt"
  Gain15/1 -> Terminator/1
  Eingabe i_GET und n_max_Upmin Spreizung 7,8/1(BUS OUT) -> Multiport Switch2/2
  Constant11/1 -> Multiport Switch2/1, Display1/1  "auswahl_getriebe"
  Eingabe i_GET und n_max_Upmin Spreizung 7,0/1(BUS OUT) -> Multiport Switch2/3
  Eingabe i_GET und n_max_Upmin Andere Angaben/1(BUS OUT) -> Multiport Switch2/5
  Eingabe i_GET und n_max_Upmin Audi RS3 8YA PA/1(BUS OUT) -> Multiport Switch2/4
  Gain17/1 -> Multiport Switch1/1  "Auswahl iAG"
  Constant13/1 -> Multiport Switch1/2
  Constant14/1 -> Multiport Switch1/3
  Constant12/1 -> Gain17/1, Display2/1  "auswahl_uebersetzung_achsgetriebe"
  Constant21/1 -> Multiport Switch1/6
  Constant20/1 -> Multiport Switch1/5
  Constant15/1 -> Multiport Switch1/4
  Constant25/1 -> Gain12/1
  Gain19/1 -> Bus Creator2/2  "Auswahl EM VA"
  Gain18/1 -> Bus Creator2/1  "Auswahl VKM"
  Gain20/1 -> Bus Creator2/3  "Auswahl EM HA"
  Constant17/1 -> Display5/1, Gain19/1  "auswahl_kennlinie_EM_P2"
  Constant19/1 -> Display6/1, Gain20/1  "auswahl_kennlinie_EM_P4"
  Constant16/1 -> Display4/1, Gain18/1  "auswahl_kennlinie_VKM"
  Constant18/1 -> Display3/1  "cp_Zelle_JpkgK"
  Constant10/1 -> Display/1  "T_init_degC"
  Constant28/1 -> Gain10/1

== system Simulation_Fahrmodell_v3_straight_line_R2024b/Vehicle Properties/Systemkonstanten ==
  BIT WHEEL BAS : Constant  OutDataTypeStr=int32
  BIT WHEEL CHAL : Constant  OutDataTypeStr=int32
  Bus Creator : BusCreator  Inputs=11
  Fahrprofil Auswahl : Constant  Value=24  OutDataTypeStr=int32
  Fahrzeugauswahl_BASIS_Fahrzeug : Constant  Value=2
  Fahrzeugauswahl_CHALLENGER : Constant  Value=7
  PHEV VAR ENG : Constant  Value=3  OutDataTypeStr=int32
  SKO FAHRER : Constant  Value=5.059393274853801  OutDataTypeStr=double
  SKO_STREET_BAS : Constant  Value=2  OutDataTypeStr=int32
  SKO_STREET_CHAL : Constant  Value=SKO_STREET_CHAL  OutDataTypeStr=int32
  SKO_STREET_CHAL1 : Constant  OutDataTypeStr=int32
  SKO_WHEEL_TYP_BAS : Constant  Value=2  OutDataTypeStr=int32
  SKO_WHEEL_TYP_CHAL : Constant  Value=SKO_WHEEL_TYP_CHAL  OutDataTypeStr=int32
  SKO_WHEEL_TYP_CHAL1 : Constant  Value=4  OutDataTypeStr=int32
  M_BUS_SKO : Outport
  wires:
  Bus Creator/1 -> M_BUS_SKO/1
  SKO_WHEEL_TYP_CHAL/1 -> Bus Creator/10  "SKO_WHEEL_TYP_CHAL"
  SKO_WHEEL_TYP_BAS/1 -> Bus Creator/7  "SKO_WHEEL_TYP_BAS"
  Fahrzeugauswahl_BASIS_Fahrzeug/1 -> Bus Creator/1  "TYP_SKO_BAS"
  Fahrzeugauswahl_CHALLENGER/1 -> Bus Creator/2  "TYP_SKO_CHAL"
  SKO FAHRER/1 -> Bus Creator/5  "SKO_BRAKE"
  SKO_STREET_CHAL/1 -> Bus Creator/11  "SKO_STREET_CHAL"
  SKO_STREET_BAS/1 -> Bus Creator/8  "SKO_STREET_BAS"
  BIT WHEEL BAS/1 -> Bus Creator/6  "SKO BIT  WHEEL BAS"
  BIT WHEEL CHAL/1 -> Bus Creator/9  "SKO BIT WHEEL CHAL"
  PHEV VAR ENG/1 -> Bus Creator/4  "SKO PHEV VAR ENG"
  Fahrprofil Auswahl/1 -> Bus Creator/3  "SKO_Fahrprofil"

== system Simulation_Fahrmodell_v3_straight_line_R2024b/Env/Nürburgring (M. Siesmann)/Fahrdynamik: Kurvenradius und Querbeschleunigung ==
  v_ist_kmph : Inport
  s_m : Inport  Port=2
  "Betrag ziehen, da links/rechts unwichtig" : Abs  SaturateOnIntegerOverflow=off
  Divide : Product  Inputs=*/
  Gain3 : Gain  Gain=1/3.6
  Product : Product
  R__m(s_cum_m) : Lookup_n-D  Commented=through  NumberOfTableDimensions=1  BreakpointsForDimension1=Track.RoundOnly.s_cum__m  Table=Track.RoundOnly.R__m  InternalRulePriority=Speed  RndMeth=Simplest
  a_y_ist_mps2 : Outport
  r_kurven_m : Outport  Port=2
  wires:
  Divide/1 -> a_y_ist_mps2/1  "a_y_ist_mps2"
  Gain3/1 -> Product/2, Product/1
  R__m(s_cum_m)/1 -> "Betrag ziehen, da links/rechts unwichtig"/1  "r_kurven_m"
  s_m/1 -> R__m(s_cum_m)/1
  Product/1 -> Divide/1  "v_ist_mps ^ 2"
  v_ist_kmph/1 -> Gain3/1
  "Betrag ziehen, da links/rechts unwichtig"/1 -> r_kurven_m/1, Divide/2

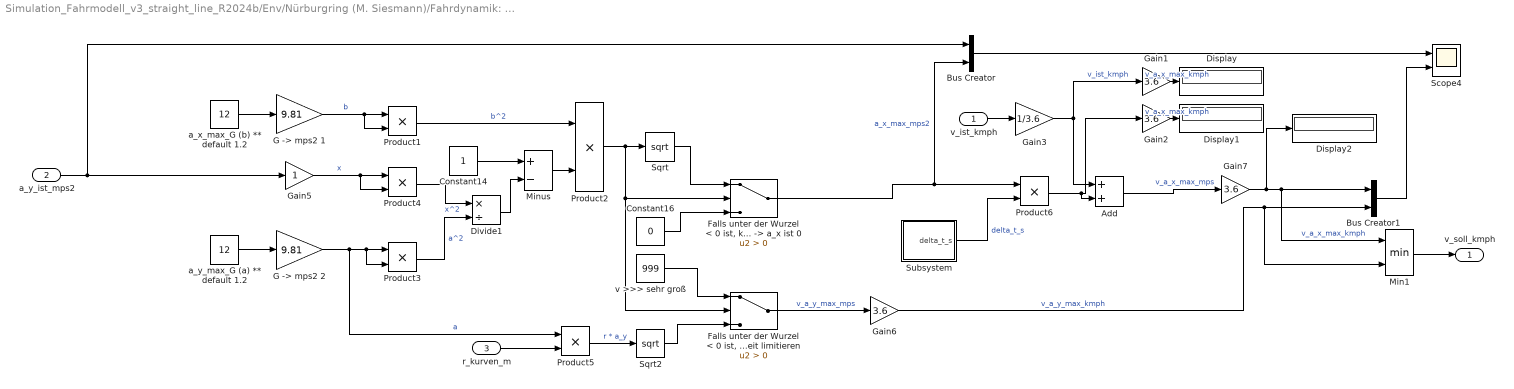
== system Simulation_Fahrmodell_v3_straight_line_R2024b/Env/Nürburgring (M. Siesmann)/Fahrdynamik: Sollgeschwindigkeit (Kamm'scher Kreis) ==
  v_ist_kmph : Inport
  a_y_ist_mps2 : Inport  Port=2
  r_kurven_m : Inport  Port=3
  Add : Sum
  Bus Creator : BusCreator  Inputs=2
  Bus Creator1 : BusCreator  Inputs=2
  Constant14 : Constant
  Constant16 : Constant  Value=0
  Display : Display
  Display1 : Display
  Display2 : Display
  Divide1 : Product  Inputs=*/
  "Falls unter der Wurzel < 0 ist, kein Potenzial in x Richtung -> a_x ist 0" : Switch  Criteria=u2 > Threshold  SaturateOnIntegerOverflow=off  InputSameDT=off
  "Falls unter der Wurzel < 0 ist, max. Geschwindigkeit limitieren -> Geschwindigkeit limitieren" : Switch  Criteria=u2 > Threshold  SaturateOnIntegerOverflow=off  InputSameDT=off
  "G -> mps2 1" : Gain  Gain=9.81
  "G -> mps2 2" : Gain  Gain=9.81
  Gain{1..2,6..7} (4 alike) : Gain  Gain=3.6
  Gain3 : Gain  Gain=1/3.6
  Gain5 : Gain
  Min1 : MinMax  Inputs=2
  Minus : Sum  Inputs=+-
  Product{1..6} (6 alike) : Product
  Scope4 : Scope  NumInputPorts=2
  Sqrt : Sqrt
  Sqrt2 : Sqrt
  Subsystem : Subsystem
  a_x_max_G (b) ** default 1.2 : Constant  Value=12
  a_y_max_G (a) ** default 1.2 : Constant  Value=12
  v >>> sehr groß : Constant  Value=999
  v_soll_kmph : Outport
  wires:
  a_x_max_G (b) ** default 1.2/1 -> "G -> mps2 1"/1
  Gain7/1 -> Min1/1, Bus Creator1/1, Display2/1  "v_a_x_max_kmph"
  Product2/1 -> "Falls unter der Wurzel < 0 ist, max. Geschwindigkeit limitieren -> Geschwindigkeit limitieren"/2, "Falls unter der Wurzel < 0 ist, kein Potenzial in x Richtung -> a_x ist 0"/2, Sqrt/1
  Minus/1 -> Product2/2
  Product4/1 -> Divide1/1  "x^2"
  Divide1/1 -> Minus/2
  Constant14/1 -> Minus/1
  "G -> mps2 2"/1 -> Product5/1, Product3/2, Product3/1  "a"
  "G -> mps2 1"/1 -> Product1/2, Product1/1  "b"
  "Falls unter der Wurzel < 0 ist, max. Geschwindigkeit limitieren -> Geschwindigkeit limitieren"/1 -> Gain6/1  "v_a_y_max_mps"
  v >>> sehr groß/1 -> "Falls unter der Wurzel < 0 ist, max. Geschwindigkeit limitieren -> Geschwindigkeit limitieren"/1
  Product3/1 -> Divide1/2  "a^2"
  a_y_max_G (a) ** default 1.2/1 -> "G -> mps2 2"/1
  Gain6/1 -> Min1/2, Bus Creator1/2  "v_a_y_max_kmph"
  Min1/1 -> v_soll_kmph/1
  Sqrt2/1 -> "Falls unter der Wurzel < 0 ist, max. Geschwindigkeit limitieren -> Geschwindigkeit limitieren"/3
  Product1/1 -> Product2/1  "b^2"
  Constant16/1 -> "Falls unter der Wurzel < 0 ist, kein Potenzial in x Richtung -> a_x ist 0"/3
  Product6/1 -> Gain2/1, Add/2
  a_y_ist_mps2/1 -> Bus Creator/1, Gain5/1
  Bus Creator1/1 -> Scope4/2
  Subsystem/1(delta_t_s) -> Product6/2  "delta_t_s"
  Add/1 -> Gain7/1  "v_a_x_max_mps"
  Product5/1 -> Sqrt2/1  "r * a_y"
  "Falls unter der Wurzel < 0 ist, kein Potenzial in x Richtung -> a_x ist 0"/1 -> Product6/1, Bus Creator/2  "a_x_max_mps2"
  Sqrt/1 -> "Falls unter der Wurzel < 0 ist, kein Potenzial in x Richtung -> a_x ist 0"/1
  Bus Creator/1 -> Scope4/1
  Gain5/1 -> Product4/2, Product4/1  "x"
  r_kurven_m/1 -> Product5/2
  v_ist_kmph/1 -> Gain3/1
  Gain3/1 -> Add/1, Gain1/1  "v_ist_kmph"
  Gain1/1 -> Display/1  "v_a_x_max_kmph"
  Gain2/1 -> Display1/1  "v_a_x_max_kmph"

== system Simulation_Fahrmodell_v3_straight_line_R2024b/Env/Nürburgring (M. Siesmann)/v max min ==
  In1 : Inport
  Constant1 : Constant  Value=1000
  Constant12 : Constant  Value=280
  Constant13 : Constant  Value=0.1
  vmax : MinMax  Inputs=2
  vmin : MinMax  Function=max  Inputs=2
  Out1 : Outport
  wires:
  vmin/1 -> Out1/1
  Constant13/1 -> vmin/1
  In1/1 -> vmax/2
  Constant1/1 -> vmax/1
  vmax/1 -> vmin/2

== system Simulation_Fahrmodell_v3_straight_line_R2024b/KPIs/time_0_to_100/Triggered Subsystem ==
  In1 : Inport
  Trigger : TriggerPort  TriggerTime=on sample time hit  VariantControl=(inherit)
  Out1 : Outport
  wires:
  In1/1 -> Out1/1

== system Simulation_Fahrmodell_v3_straight_line_R2024b/KPIs/time_0_to_200/Triggered Subsystem ==
  In1 : Inport
  Trigger : TriggerPort  TriggerTime=on sample time hit  VariantControl=(inherit)
  Out1 : Outport
  wires:
  In1/1 -> Out1/1

== system Simulation_Fahrmodell_v3_straight_line_R2024b/KPIs/time_60_to_120/time_0_to_120 ==
  In1 : Inport
  Clock : Clock
      settings: Decimation=100
  Constant : Constant
  Constant1 : Constant  Value=0
  Switch : Switch  Threshold=120  SaturateOnIntegerOverflow=off  InputSameDT=off
  Triggered Subsystem : Subsystem  TreatAsAtomicUnit=on
  Out1 : Outport
  wires:
  Constant/1 -> Switch/1
  In1/1 -> Switch/2
  Switch/1 -> Triggered Subsystem/Trigger
  Clock/1 -> Triggered Subsystem/1(In1)
  Constant1/1 -> Switch/3
  Triggered Subsystem/1(Out1) -> Out1/1

== system Simulation_Fahrmodell_v3_straight_line_R2024b/KPIs/time_60_to_120/time_0_to_60 ==
  In1 : Inport
  Clock : Clock
      settings: Decimation=100
  Constant : Constant
  Constant1 : Constant  Value=0
  Switch : Switch  Threshold=60  SaturateOnIntegerOverflow=off  InputSameDT=off
  Triggered Subsystem : Subsystem  TreatAsAtomicUnit=on
  Out1 : Outport
  wires:
  Triggered Subsystem/1(Out1) -> Out1/1
  Constant1/1 -> Switch/3
  Clock/1 -> Triggered Subsystem/1(In1)
  Switch/1 -> Triggered Subsystem/Trigger
  In1/1 -> Switch/2
  Constant/1 -> Switch/1

== system Simulation_Fahrmodell_v3_straight_line_R2024b/KPIs/time_80_to_120/time_0_to_120 ==
  In1 : Inport
  Clock : Clock
      settings: Decimation=100
  Constant : Constant
  Constant1 : Constant  Value=0
  Switch : Switch  Threshold=120  SaturateOnIntegerOverflow=off  InputSameDT=off
  Triggered Subsystem : Subsystem  TreatAsAtomicUnit=on
  Out1 : Outport
  wires:
  Triggered Subsystem/1(Out1) -> Out1/1
  Constant1/1 -> Switch/3
  Clock/1 -> Triggered Subsystem/1(In1)
  Switch/1 -> Triggered Subsystem/Trigger
  In1/1 -> Switch/2
  Constant/1 -> Switch/1

== system Simulation_Fahrmodell_v3_straight_line_R2024b/KPIs/time_80_to_120/time_0_to_80 ==
  In1 : Inport
  Clock : Clock
      settings: Decimation=100
  Constant : Constant
  Constant1 : Constant  Value=0
  Switch : Switch  Threshold=80  SaturateOnIntegerOverflow=off  InputSameDT=off
  Triggered Subsystem : Subsystem  TreatAsAtomicUnit=on
  Out1 : Outport
  wires:
  Constant/1 -> Switch/1
  In1/1 -> Switch/2
  Switch/1 -> Triggered Subsystem/Trigger
  Clock/1 -> Triggered Subsystem/1(In1)
  Constant1/1 -> Switch/3
  Triggered Subsystem/1(Out1) -> Out1/1

== system Simulation_Fahrmodell_v3_straight_line_R2024b/Vehicle Dynamics Model /Drivetrain/Axle Load and Torque Distribution  ==
  Gradient : Inport
  <S_BUS_d_wheel_CHAL> : Inport  Port=2
  acceleration : Inport  Port=3
  F_Haftgrenze [N] : Inport  Port=4
  Tq_Primary_axle : Inport  Port=5
  Tq_Secondary_axle : Inport  Port=6
  "Axle Torque Channel Router " : Subsystem
  Berechnung Max. Radlast VA/HA aufgrund Reifen/Fahrbahn : Subsystem
  Berechnung Achslastverteilung abh. Fahrzeugeigenschaften (Haken Abs. 11) : Subsystem
  Display5 : Display
  Display6 : Display
  "Drive Topology Axle Load Distributor " : Subsystem
  Subsystem : Subsystem
  Tq_max_FrontAxle_OUT : Outport
  M_HA_Nm OUT : Outport  Port=2
  wires:
  Tq_Secondary_axle/1 -> "Axle Torque Channel Router "/2(Tq_Secondary_axle)
  Berechnung Achslastverteilung abh. Fahrzeugeigenschaften (Haken Abs. 11)/1(axle_load_FrontAxle [%]) -> "Drive Topology Axle Load Distributor "/1(axle_load_FrontAxle [%]), Berechnung Max. Radlast VA/HA aufgrund Reifen/Fahrbahn/3(axle_load_FrontAxle [%])
  Berechnung Achslastverteilung abh. Fahrzeugeigenschaften (Haken Abs. 11)/2(axle_load_RearAxle [%]) -> "Drive Topology Axle Load Distributor "/2(axle_load_RearAxle [%]), Berechnung Max. Radlast VA/HA aufgrund Reifen/Fahrbahn/4(axle_load_RearAxle [%])
  "Drive Topology Axle Load Distributor "/2(M_HA_Nm OUT) -> M_HA_Nm OUT/1
  Tq_Primary_axle/1 -> "Axle Torque Channel Router "/1(Tq_Primary_axle)
  "Drive Topology Axle Load Distributor "/1(M_VA_Nm OUT) -> Tq_max_FrontAxle_OUT/1
  Gradient/1 -> Berechnung Achslastverteilung abh. Fahrzeugeigenschaften (Haken Abs. 11)/1(Steigung)
  acceleration/1 -> Berechnung Achslastverteilung abh. Fahrzeugeigenschaften (Haken Abs. 11)/2(Beschleunigung)
  F_Haftgrenze [N]/1 -> Berechnung Max. Radlast VA/HA aufgrund Reifen/Fahrbahn/1(F_Haftgrenze [N])
  <S_BUS_d_wheel_CHAL>/1 -> Berechnung Max. Radlast VA/HA aufgrund Reifen/Fahrbahn/2(Raddurchmesser [m])
  Subsystem/2(Tq_max_RearAxle) -> "Drive Topology Axle Load Distributor "/4(Tq_max_RearAxle), Display6/1
  Subsystem/1(Tq_max_FrontAxle) -> "Drive Topology Axle Load Distributor "/3(Tq_max_FrontAxle), Display5/1
  Berechnung Max. Radlast VA/HA aufgrund Reifen/Fahrbahn/1(Max. Radlast VA [Nm] aufgrund Reifen/Fahrbahn) -> Subsystem/1(In1)
  Berechnung Max. Radlast VA/HA aufgrund Reifen/Fahrbahn/2(Max. Radlast HA [Nm] aufgrund Reifen/Fahrbahn) -> Subsystem/2(In2)
  "Axle Torque Channel Router "/1(Tq_FrontAxle) -> Subsystem/3("Tq_FrontAxle ")
  "Axle Torque Channel Router "/2(Tq_RearAxle) -> Subsystem/4("Tq_RearAxle ")

== system Simulation_Fahrmodell_v3_straight_line_R2024b/Vehicle Dynamics Model /Drivetrain/Berechnung Leistung 1 ==
  F_N : Inport
  v_mps : Inport  Port=2
  Product : Product
  "W -> kW" : Gain  Gain=0.001
  P_kW : Outport
  wires:
  F_N/1 -> Product/1
  v_mps/1 -> Product/2
  Product/1 -> "W -> kW"/1
  "W -> kW"/1 -> P_kW/1

== system Simulation_Fahrmodell_v3_straight_line_R2024b/Vehicle Dynamics Model /Drivetrain/Betriebsstrategie mit motorseitigen Leistungen ==
  P_ges_kW : Inport
  P_max_VKM_kW : Inport  Port=2
  P_min_VKM_kW : Inport  Port=3
  P_max_EM_P2_kW : Inport  Port=4
  P_min_EM_P2_kW : Inport  Port=5
  Add : Sum
  Add1 : Sum
  Bus Creator : BusCreator  Inputs=2
  Bus Creator1 : BusCreator  Inputs=2
  Constant : Constant  Value=0
  Constant1 : Constant  Value=0
  Display : Display
  Max : MinMax  Function=max  Inputs=2
  Max1 : MinMax  Inputs=2
  Min1 : MinMax  Inputs=2
  Min2 : MinMax  Function=max  Inputs=2
  Min3 : MinMax  Function=max  Inputs=2
  Min4 : MinMax  Inputs=2
  Minus1 : Sum  Inputs=+-
  Minus2 : Sum  Inputs=+-
  Minus4 : Sum  Inputs=+-
  Scope : Scope  NumInputPorts=4
  Scope1 : Scope  NumInputPorts=3
  Scope2 : Scope
  Scope3 : Scope  NumInputPorts=3
  P_VKM_kW : Outport
  P_EM_kW : Outport  Port=2
  P_Bremse_kW : Outport  Port=3
  wires:
  Minus4/1 -> Min1/1
  P_max_EM_P2_kW/1 -> Min1/2, Bus Creator1/1  "P_max_EM_P2_kW"
  Min1/1 -> Add1/1
  Constant/1 -> Max/2
  Max/1 -> Min4/1, Minus4/1
  P_ges_kW/1 -> Scope/1, Scope1/1, Max1/1, Max/1, Scope3/1  "P_ges_kW"
  Constant1/1 -> Max1/2
  Max1/1 -> Minus2/1, Min2/1
  P_min_VKM_kW/1 -> Min2/2, Bus Creator/2  "P_min_VKM_kW"
  Min2/1 -> Scope1/2, Add/2, Minus2/2
  Add/1 -> Scope/2, P_VKM_kW/1  "P_VKM_kW"
  Minus2/1 -> Minus1/1, Min3/1
  P_min_EM_P2_kW/1 -> Scope2/1, Min3/2, Bus Creator1/2  "P_min_EM_P2_kW"
  Add1/1 -> Scope/3, Display/1, P_EM_kW/1  "P_EM_kW"
  Min3/1 -> Scope1/3, Add1/2, Minus1/2
  Min4/1 -> Add/1, Minus4/2
  Minus1/1 -> P_Bremse_kW/1, Scope/4  "P_Bremse_kW"
  P_max_VKM_kW/1 -> Bus Creator/1, Min4/2  "P_max_VKM_kW"
  Bus Creator/1 -> Scope3/2
  Bus Creator1/1 -> Scope3/3
